simulink model "Kalman_FSFB_Sim"  (R2019b)
settings: Solver=VariableStepAuto  StartTime=0.0  StopTime=30  RelTol=1e-3
values from neighbouring files (symbols this model uses):
  A = [0 1; -2 3]    [Kalman_FSFB.m]    (also in LQR_MSD.m = [0      1)
  B = [0 1]'    [Kalman_FSFB.m]    (also in LQR_MSD.m = [0)
  B1 = [2 1]'    [Kalman_FSFB.m]
  C = [1 1]    [Kalman_FSFB.m]    (also in LQR_MSD.m = eye(2))
  D = [1]    [Kalman_FSFB.m]    (also in LQR_MSD.m = [0)
  K = lqr(A,B1,eye(2),0.25)    [Kalman_FSFB.m]
  L = P*C'/(D*D')    [Kalman_FSFB.m]
libraries: simulink x4
settings Model: Creator=bala4krish  LastModifiedBy=bala4krish
settings DataIOCC: ReturnWorkspaceOutputs=off

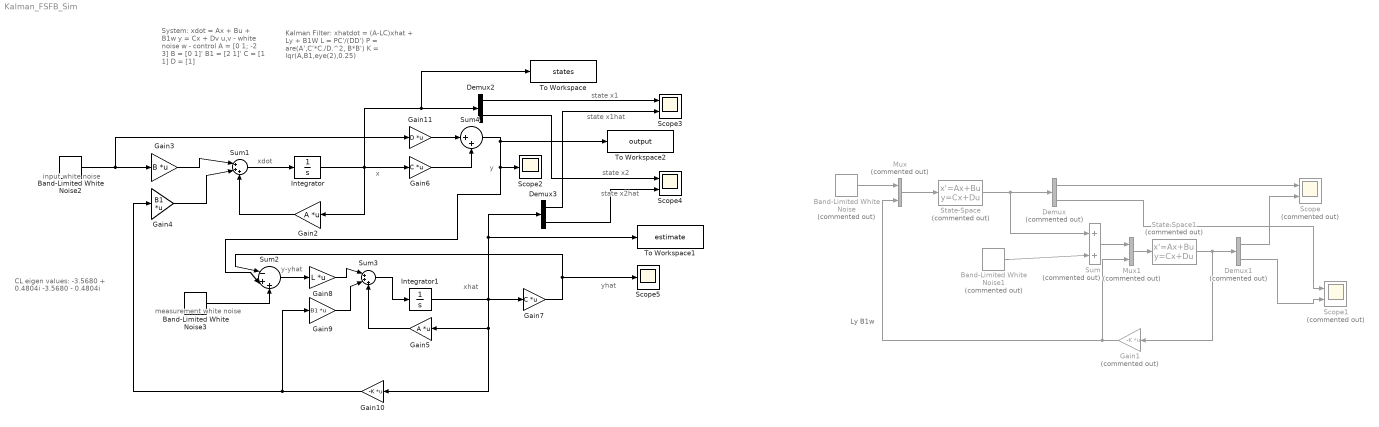
== system Kalman_FSFB_Sim ==
  note: xdot
  note: System:
      |
      | xdot = Ax + Bu + B1w
      | y = Cx + Dv
      | u,v - white noise
      | w - control
      |
      | A = [0 1; -2 3]
      | B = [0 1]'
      | B1 = [2 1]'
      | C = [1 1]
      | D = [1]
  note: state x1hat
  note: state x1
  note: measurement white noise
  note: input white noise
  note: y-yhat
  note: xhat
  note: y
  note: x
  note: yhat
  note: Ly
      | B1w
  note: Kalman Filter:
      |
      | xhatdot = (A-LC)xhat + Ly + B1W
      | L = PC'/(DD')
      | P = are(A',C'*C./D.^2, B*B')
      | K = lqr(A,B1,eye(2),0.25)
  note: state x2hat
  note: state x2
  note: CL eigen values:
      |
      | -3.5680 + 0.4804i
      | -3.5680 - 0.4804i
  Band-Limited White Noise : simulink/Sources/Band-Limited White Noise  Commented=on  Cov=0.1  Ts=0.1  seed=[23341]
  Band-Limited White Noise1 : simulink/Sources/Band-Limited White Noise  Commented=on  Cov=0.1  Ts=0.1  seed=[23342]
  Band-Limited White Noise2 : simulink/Sources/Band-Limited White Noise  Cov=0.1  Ts=0.1  seed=[23341]
  Band-Limited White Noise3 : simulink/Sources/Band-Limited White Noise  Cov=0.1  Ts=0.1  seed=[23342]
  Demux : Demux  Commented=on  Outputs=2
  Demux1 : Demux  Commented=on  Outputs=2
  Demux2 : Demux  Outputs=2
  Demux3 : Demux  Outputs=2
  Gain1 : Gain  Commented=on  Gain=-K  Multiplication=Matrix(K*u)
  Gain10 : Gain  Gain=-K  Multiplication=Matrix(K*u)
  Gain11 : Gain  Gain=D  Multiplication=Matrix(K*u)
  Gain2 : Gain  Gain=A  Multiplication=Matrix(K*u)
  Gain3 : Gain  Gain=B  Multiplication=Matrix(K*u)
  Gain4 : Gain  Gain=B1  Multiplication=Matrix(K*u)
  Gain5 : Gain  Gain=A  Multiplication=Matrix(K*u)
  Gain6 : Gain  Gain=C  Multiplication=Matrix(K*u)
  Gain7 : Gain  Gain=C  Multiplication=Matrix(K*u)
  Gain8 : Gain  Gain=L  Multiplication=Matrix(K*u)
  Gain9 : Gain  Gain=B1  Multiplication=Matrix(K*u)
  Integrator : Integrator
  Integrator1 : Integrator
  Mux : Mux  Commented=on  Inputs=2
  Mux1 : Mux  Commented=on  Inputs=2
  Scope : Scope  Commented=on  NumInputPorts=2
  Scope1 : Scope  Commented=on  NumInputPorts=2
  Scope2 : Scope
  Scope3 : Scope  NumInputPorts=2
  Scope4 : Scope  NumInputPorts=2
  Scope5 : Scope
  State-Space : StateSpace  Commented=on  A=A  B=B  C=C  D=[1;1];  InitialCondition=0
  State-Space1 : StateSpace  Commented=on  A=A-L*C  B=[L B1]  C=C  D=[1 1]  InitialCondition=0
  Sum : Sum  Commented=on  Inputs=|++
  Sum1 : Sum  Inputs=|+++
  Sum2 : Sum  Inputs=|-++
  Sum3 : Sum  Inputs=|+++
  Sum4 : Sum  Inputs=|++
  To Workspace : ToWorkspace  VariableName=states  SaveFormat=Structure With Time  SampleTime=-1
  To Workspace1 : ToWorkspace  VariableName=estimate  SaveFormat=Structure With Time  SampleTime=-1
  To Workspace2 : ToWorkspace  VariableName=output  SaveFormat=Structure With Time  SampleTime=-1
  wires:
  Band-Limited White Noise/1 -> Mux/1
  Mux/1 -> State-Space/1
  State-Space/1 -> Demux/1, Sum/1
  Mux1/1 -> State-Space1/1
  State-Space1/1 -> Demux1/1, Gain1/1
  Demux1/2 -> Scope1/2
  Gain1/1 -> Mux/2, Mux1/2
  Sum/1 -> Mux1/1
  Demux/2 -> Scope1/1
  Band-Limited White Noise1/1 -> Sum/2
  Demux/1 -> Scope/1
  Demux1/1 -> Scope/2
  Integrator/1 -> Gain2/1, To Workspace/1, Demux2/1, Gain6/1
  Gain2/1 -> Sum1/3
  Band-Limited White Noise2/1 -> Gain11/1, Gain3/1
  Gain3/1 -> Sum1/1
  Gain4/1 -> Sum1/2
  Sum1/1 -> Integrator/1
  Gain5/1 -> Sum3/3
  Sum3/1 -> Integrator1/1
  Integrator1/1 -> Gain5/1, Gain10/1, Demux3/1, To Workspace1/1, Gain7/1
  Sum4/1 -> To Workspace2/1, Sum2/2, Scope2/1
  Band-Limited White Noise3/1 -> Sum2/3
  Sum2/1 -> Gain8/1
  Gain8/1 -> Sum3/1
  Gain9/1 -> Sum3/2
  Gain7/1 -> Scope5/1, Sum2/1
  Gain10/1 -> Gain9/1, Gain4/1
  Demux2/1 -> Scope3/1
  Demux3/1 -> Scope3/2
  Demux3/2 -> Scope4/2
  Demux2/2 -> Scope4/1
  Gain11/1 -> Sum4/1
  Gain6/1 -> Sum4/2
